simulink model "DFT_Ex5"  (R2023a)
settings: Solver=VariableStepAuto  StartTime=0.0  StopTime=0.1  RelTol=1e-3
StartFcn:
  | FramesPerWindow = 2;
undefined symbols (not defined in the file): None, S, vsva2197, xcvc1902
libraries: aieUtilities x2, dspsrcs4 x1, aieDSP x1, vmcUtilities x1
settings Model: Creator=sdegala  LastModifiedBy=robg
settings ModelReferenceCC: EnableRefExpFcnMdlSchedulingChecks=on

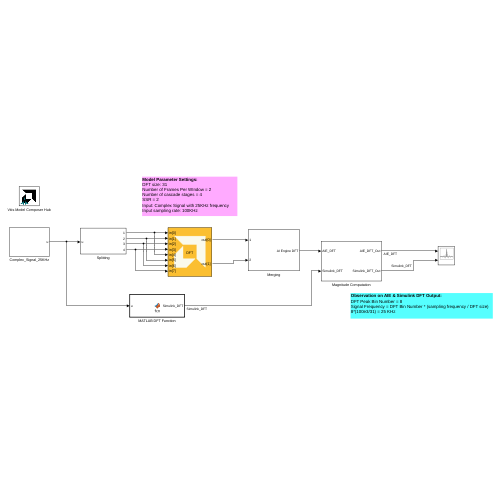
[thumbnail: Simulink's stored preview of the top-level diagram]
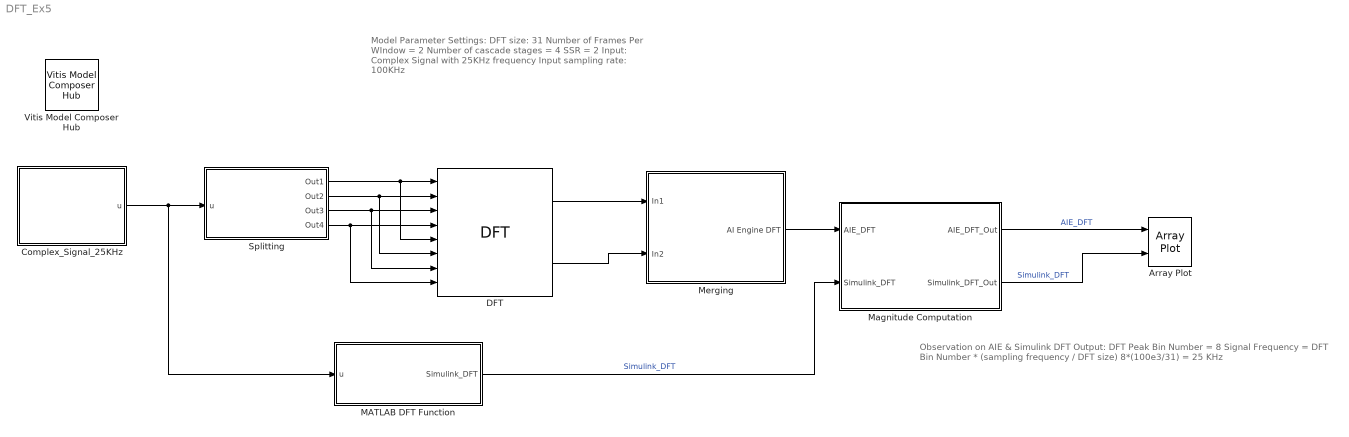
== system DFT_Ex5 ==
  note: Model Parameter Settings:
      | DFT size: 31
      | Number of Frames Per WIndow = 2
      | Number of cascade stages = 4
      | SSR = 2
      | Input: Complex Signal with 25KHz frequency
      | Input sampling rate: 100KHz
  note: Observation on AIE & Simulink DFT Output:
      | DFT Peak Bin Number = 8
      | Signal Frequency = DFT Bin Number * (sampling frequency / DFT size)
      | 8*(100e3/31) = 25 KHz
  Array Plot : ArrayPlot  NumInputPorts=2  WindowPosition=[1.000000,1.000000,1280.000000,744.000000,]  Visible=on  ScopeFrameLocation=window  YLimits=[-36.25 346.25]  ShowLegend=on
  Complex_Signal_25KHz : Subsystem
  DFT : aieDSP/DFT  data_type=cint16  twiddle_type=cint16  point_size=31  num_frames=2  shift_val=0  rnd_mode=Floor  ssr=2  sat_mode=0-None  casc_length=4  AIE_VARIANT=1  blockJsonConstraints=[]  blockJsonConstraintsInternal=[]  spec=vmc_dft.json  SerializedMaskParamNames=[]  SerializedMaskParamValues=[]  SerializedMaskParamVisibilities=[]  block_type=DFT  SerializedMaskParamDataypes=typename|typename|uint|uint|uint|uint|uint|uint|uint|uint  SerializedMaskParamEnumStrArr=0|0|0|0|0|Floor,Ceiling,Round to positive infinity,Round to negative infinity,Round symmetrical to infinity,Round symmetrical to zero,Round convergent to even,Round convergent to odd|0|0-None,1-Asymmetric,3-Symmetric|0|0  SerializedMaskParamEnumValArr=0|0|0|0|0|0,1,2,3,4,5,6,7|0|0,1,3|0|0  SerializedMaskParamVectorArr=0|0|0|0|0|0|0|0|0|0
  MATLAB DFT Function : MATLAB Function  TreatAsAtomicUnit=on
  Magnitude Computation : Subsystem
  Merging : Subsystem
  Splitting : Subsystem
  Vitis Model Composer Hub : vmcUtilities/Vitis Model Composer Hub  Tag=genX  CodeGeneration=off  StartColumn=1  NumberOfColumns=1  TargetDirectory=./code  exportDesign=off  analyzeDesign=off  validateDesignOnHw=off  ExportType=AI Engines  IpVendor=xilinx.com  IpLibrary=hls  IpVersion=1.0  IpHWLanguage=Verilog  AieCompilerOptions={}  AieSimulatorOptions={}  CreateTestbench=off  TestbenchStackSize=10  RunRtlSim=off  RunCSim=off  RunAieSim=off  AieSimTimeout=50000  RunAieSimProfiling=off  LaunchVitisAnalyzer=off  PlotOutput=off  RunX86Sim=off  X86SimTimeout=10  GenHwImage=off  GenLibadfXo=off  GenHwValidationCode=off  PlatformType=Not Specified  HwSystemType=Baremetal  HwValidationTarget=hw  ProjDevice=xcvc1902-vsva2197-1LP-e-S  ProjDevicePart=xcvc1902-vsva2197-1LP-e-S  AIEType=AIE  SamplePeriod=-1  ClockFrequency=200  DataPathParallelism=1  xilinxfamily=versalaicore  part=xcvc1902  speed=-1LP-e-S  package=vsva2197  directory=./code  testbench=off  incr_netlist=off  synthesis_tool=Vivado  clock_wrapper=Clock Enables  dbl_ovrd=According to Block Masks  dcm_input_clock_period=10  sysclk_period=10  simulink_period=1  eval_field=0  LogFileName=''  NThreads=4
  wires:
  Complex_Signal_25KHz/1(u) -> MATLAB DFT Function/1(u), Splitting/1(u)
  Magnitude Computation/1(AIE_DFT_Out) -> Array Plot/1  "AIE_DFT"
  Magnitude Computation/2(Simulink_DFT_Out) -> Array Plot/2  "Simulink_DFT"
  Splitting/1(Out1) -> DFT/5, DFT/1
  Splitting/2(Out2) -> DFT/6, DFT/2
  Splitting/3(Out3) -> DFT/7, DFT/3
  Splitting/4(Out4) -> DFT/8, DFT/4
  MATLAB DFT Function/1(Simulink_DFT) -> Magnitude Computation/2(Simulink_DFT)  "Simulink_DFT"
  DFT/1 -> Merging/1(In1)
  DFT/2 -> Merging/2(In2)
  Merging/1(AI Engine DFT) -> Magnitude Computation/1(AIE_DFT)

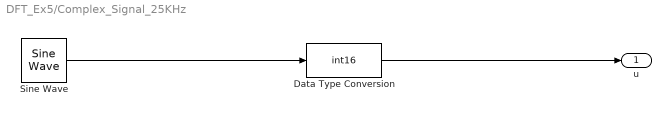
== system DFT_Ex5/Complex_Signal_25KHz ==
  Data Type Conversion : DataTypeConversion  OutDataTypeStr=int16  ConvertRealWorld=Stored Integer (SI)  SaturateOnIntegerOverflow=off  RndMeth=Floor
  Sine Wave : dspsrcs4/Sine Wave  Amplitude=1  Frequency=25e3  Phase=0  SampleMode=Discrete  OutComplex=Complex  CompMethod=Table lookup  TableSize=Speed  SampleTime=1/100e3  SamplesPerFrame=64  ResetState=Restart at time zero  OutputFrames=off  dataType=Fixed-point  wordLen=16  udDataType=sfix(16)  fracBitsMode=User-defined  numFracBits=10  OutDataTypeStr=fixdt(1,16,10)  LastOutDataTypeStr=fixdt(1,16,10)
  u : Outport
  wires:
  Data Type Conversion/1 -> u/1
  Sine Wave/1 -> Data Type Conversion/1

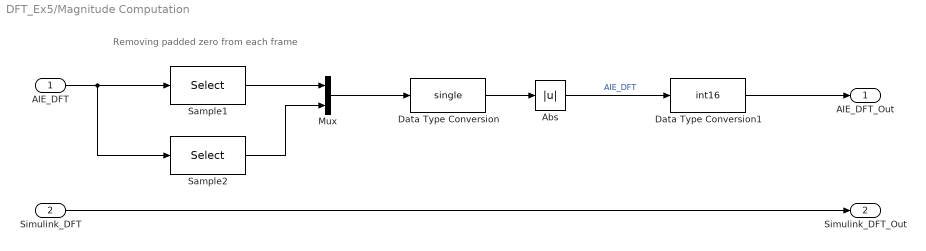
== system DFT_Ex5/Magnitude Computation ==
  note: Removing padded zero from each frame
  AIE_DFT : Inport
  Simulink_DFT : Inport  Port=2
  Abs : Abs  SaturateOnIntegerOverflow=off
  Data Type Conversion : DataTypeConversion  OutDataTypeStr=single  SaturateOnIntegerOverflow=off  RndMeth=Floor
  Data Type Conversion1 : DataTypeConversion  OutDataTypeStr=int16  SaturateOnIntegerOverflow=off  RndMeth=Floor
  Mux : Mux  Inputs=2
  Sample1 : Selector  IndexMode=Zero-based  InputPortWidth=64  IndexOptions=Index vector (dialog)  Indices=0:1:30  OutputSizes=1
  Sample2 : Selector  IndexMode=Zero-based  InputPortWidth=64  IndexOptions=Index vector (dialog)  Indices=32:1:62  OutputSizes=1
  AIE_DFT_Out : Outport
  Simulink_DFT_Out : Outport  Port=2
  wires:
  Data Type Conversion/1 -> Abs/1
  Data Type Conversion1/1 -> AIE_DFT_Out/1
  Abs/1 -> Data Type Conversion1/1  "AIE_DFT"
  Simulink_DFT/1 -> Simulink_DFT_Out/1
  AIE_DFT/1 -> Sample2/1, Sample1/1
  Sample1/1 -> Mux/1
  Sample2/1 -> Mux/2
  Mux/1 -> Data Type Conversion/1

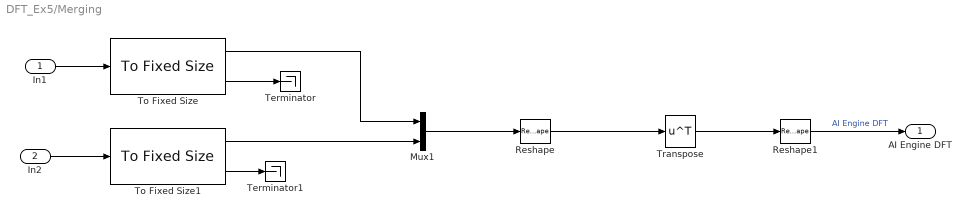
== system DFT_Ex5/Merging ==
  In1 : Inport
  In2 : Inport  Port=2
  Mux1 : Mux  Inputs=2
  Reshape : Reshape  OutputDimensionality=Customize  OutputDimensions=[32, 2]
  Reshape1 : Reshape  OutputDimensions=[1, 10]
  Terminator : Terminator
  Terminator1 : Terminator
  To Fixed Size : aieUtilities/To Fixed Size  Mode=Produce a valid output signal  OutputSize=Inherit: Same as input  CopyMethod=Buffer samples to form output  HasStatusOutput=on
  To Fixed Size1 : aieUtilities/To Fixed Size  Mode=Produce a valid output signal  OutputSize=Inherit: Same as input  CopyMethod=Buffer samples to form output  HasStatusOutput=on
  Transpose : Math  Operator=transpose
  AI Engine DFT : Outport
  wires:
  To Fixed Size1/2 -> Terminator1/1
  To Fixed Size/2 -> Terminator/1
  Transpose/1 -> Reshape1/1
  To Fixed Size1/1 -> Mux1/2
  Reshape/1 -> Transpose/1
  In1/1 -> To Fixed Size/1
  Reshape1/1 -> AI Engine DFT/1  "AI Engine DFT"
  To Fixed Size/1 -> Mux1/1
  Mux1/1 -> Reshape/1
  In2/1 -> To Fixed Size1/1

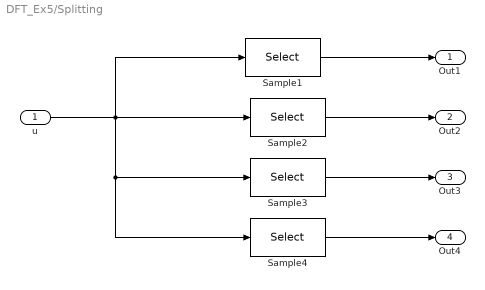
== system DFT_Ex5/Splitting ==
  u : Inport
  Sample1 : Selector  InputPortWidth=64  IndexOptions=Index vector (dialog)  Indices=1:4:64  OutputSizes=1
  Sample2 : Selector  InputPortWidth=64  IndexOptions=Index vector (dialog)  Indices=2:4:64  OutputSizes=1
  Sample3 : Selector  InputPortWidth=64  IndexOptions=Index vector (dialog)  Indices=3:4:64  OutputSizes=1
  Sample4 : Selector  InputPortWidth=64  IndexOptions=Index vector (dialog)  Indices=4:4:64  OutputSizes=1
  Out1 : Outport
  Out2 : Outport  Port=2
  Out3 : Outport  Port=3
  Out4 : Outport  Port=4
  wires:
  u/1 -> Sample4/1, Sample3/1, Sample2/1, Sample1/1
  Sample2/1 -> Out2/1
  Sample1/1 -> Out1/1
  Sample3/1 -> Out3/1
  Sample4/1 -> Out4/1

== matlab function DFT_Ex5/MATLAB DFT Function ==
  data: u input; Simulink_DFT output

function Simulink_DFT  = fcn(u)

DFT_Size = 31; % DFT Size
FramesPerWindow = 2; %No.of Frames Per Window
u = single(u);

X = single(complex(zeros(DFT_Size,FramesPerWindow)));

for m = 1:1:FramesPerWindow
for k = 0:DFT_Size-1
    for n = 0:DFT_Size-1
        X(k+1,m) = X(k+1,m) + u(n+1)*exp(-1i*2*pi*n*k/DFT_Size);
    end
end
end

Simulink_DFT = int16(abs(reshape(X,DFT_Size*FramesPerWindow,1)));
